simulink model "sfcndemo_barplot"  (Simulink 7.6)
settings: Solver=VariableStepDiscrete  StartTime=0.0  StopTime=inf  FixedStep=1  RelTol=1e-3
libraries: simulink_extras x1
Description:
  | Custom Scope (Signal Viewer) Without Wires C-MEX S-function
settings Model: Creator=The MathWorks Inc.  ExtModeTrigMode=oneshot  ExtModeArmWhenConnect=off  ExtModeAutoUpdateStatusClock=off  BufferReuse=off
settings DataIOCC: LimitDataPoints=off
settings OptimizationCC: BlockReduction=off  BooleanDataType=off  InlineInvariantSignals=on  OptimizeBlockIOStorage=off  BufferReuse=off  ExpressionFolding=off  LocalBlockOutputs=off  InitFltsAndDblsToZero=on
settings DebuggingCC: SaveWithParameterizedLinksMsg=none  SignalResolutionControl=TryResolveAllWithWarning  SolverPrmCheckMsg=none  MultiTaskDSMMsg=warning  MultiTaskCondExecSysMsg=none
settings HardwareCC: TargetUnknown=on
settings RTWCC: IncludeERTFirstTime=on
settings CodeAppCC: CustomSymbolStrFcn=$F$N$M
settings GRTTargetCC: TargetFcnLib=ansi_tfl_tmw.mat

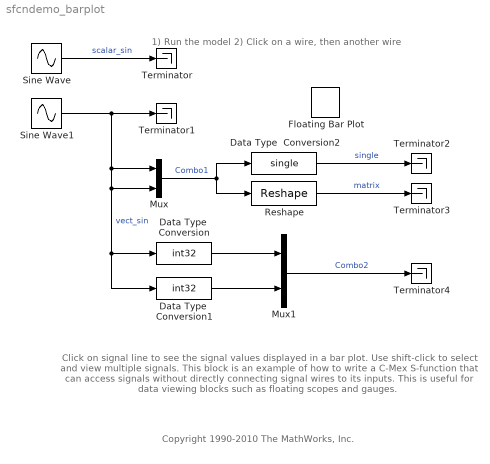
== system sfcndemo_barplot ==
  note: Click on signal line to see the signal values displayed in a bar plot.
      | Use shift-click to select and view multiple signals.
      |
      | This block is an example of how to write a C-Mex S-function that can
      | access signals without directly connecting signal wires to its inputs.  This
      | is useful for data viewing blocks such as floating scopes and gauges.
  note: Copyright 1990-2010 The MathWorks, Inc.
  note: 1) Run the model
      | 2) Click on a wire,
      |     then another wire
  Data Type  Conversion : DataTypeConversion  OutDataTypeStr=int32  SaturateOnIntegerOverflow=on  RndMeth=Zero
  Data Type  Conversion1 : DataTypeConversion  OutDataTypeStr=int32  SaturateOnIntegerOverflow=on  RndMeth=Zero
  Data Type  Conversion2 : DataTypeConversion  OutDataTypeStr=single  SaturateOnIntegerOverflow=on  RndMeth=Zero
  Floating Bar Plot : simulink_extras/Additional Sinks/Floating Bar Plot  yLim="[-6 6  -5 5  -5 5  -5 5  -5 5  -5 5  -5 5  -5 5  -5 5  -5 5  -5 5]"
  Mux : Mux  Inputs=2
  Mux1 : Mux  Inputs=2
  Reshape : Reshape  OutputDimensionality=Customize  OutputDimensions=[4,3]
  Sine Wave : Sin  SampleTime=0
  Sine Wave1 : Sin  Amplitude=1:6  Phase=[0 pi/16 pi/8 pi/4 pi/2 pi ]  SampleTime=0
  Terminator{,1..4} (5 alike) : Terminator
  wires:
  Sine Wave/1 -> Terminator/1  "scalar_sin"
  Data Type  Conversion/1 -> Mux1/1
  Data Type  Conversion1/1 -> Mux1/2
  Mux1/1 -> Terminator4/1  "Combo2"
  Sine Wave1/1 -> Terminator1/1, Mux/1, Mux/2, Data Type  Conversion/1, Data Type  Conversion1/1  "vect_sin"
  Reshape/1 -> Terminator3/1  "matrix"
  Mux/1 -> Data Type  Conversion2/1, Reshape/1  "Combo1"
  Data Type  Conversion2/1 -> Terminator2/1  "single"
